simulink model "MAS_180_BO"  (R2018b)
settings: Solver=VariableStepAuto  StartTime=0.0  StopTime=10.0  RelTol=1e-3
values from neighbouring files (symbols this model uses):
  A = sqrt(2/3)*[1 -0.5 -0.5; 0 sqrt(3)/2 -sqrt(3)/2; sqrt(0.5) sqrt(0.5) sqrt(0.5)]    [MAS_EVV_init.m]
  a1 = input('Reponse : ')    [MAS_EVV_init.m]
  Ai = inv(A)    [MAS_EVV_init.m]
  alfa = 3.98e-3    (= 0.00398)    [MAS_EVV_init.m]
  b1 = input('Reponse : ')    [MAS_EVV_init.m]
  Bi = [1/(sigma*Ls) 0 -Msr/(sigma*Ls*Lr) 0; 0 1/(sigma*Ls) 0 -Msr/(sigma*Ls*Lr); -Msr/(sigma*Ls*Lr) 0 1/(sigma*Ls) 0; 0 -Msr/(sigma*Ls*Lr) 0 1/(sigma*Ls) ]    [MAS_EVV_init.m]
  c1 = input('Reponse : ')    [MAS_EVV_init.m]
  d1 = input('Reponse : ')    [MAS_EVV_init.m]
  delta_T = 80    [MAS_EVV_init.m]
  f = (alpha/100)*Pn/(Wn)^2    (= 0.000141076783904)    [MAS_EVV_init.m]    (also in fct_trans.m)
  J = 0.51    [MAS_EVV_init.m]    (also in fct_trans.m)
  Lr = (N2w/2+L1w)/wn    [MAS_EVV_init.m]    (also in fct_trans.m)
  Ls = (N2w/2+L1w)/wn    [MAS_EVV_init.m]    (also in fct_trans.m)
  Msr = L1w/wn    [MAS_EVV_init.m]    (also in fct_trans.m)
  P = 1    [MAS_EVV_init.m]    (also in fct_trans.m)
  R0 = Rr/(1+alfa*delta_T)    [MAS_EVV_init.m]
  Rr = double(R2)    [MAS_EVV_init.m]    (also in fct_trans.m)
  Rs = 0.9*Rr    [MAS_EVV_init.m]    (also in fct_trans.m)
  sigma = 1-(Msr^2)/(Ls*Lr)    [MAS_EVV_init.m]    (also in fct_trans.m)
  to = 1    [MAS_EVV_init.m]
  variable = 1    [MAS_EVV_init.m]
  Vn = Un/sqrt(3)    [MAS_EVV_init.m]    (also in fct_trans.m)
  Wn = 2*pi*Nn/60    (= 309.342156623)    [MAS_EVV_init.m]    (also in fct_trans.m)
  wn = 2*pi*fn    (= 314.159265359)    [MAS_EVV_init.m]    (also in fct_trans.m)
settings Model: Creator=cindyiskandar  LastModifiedBy=cindyiskandar

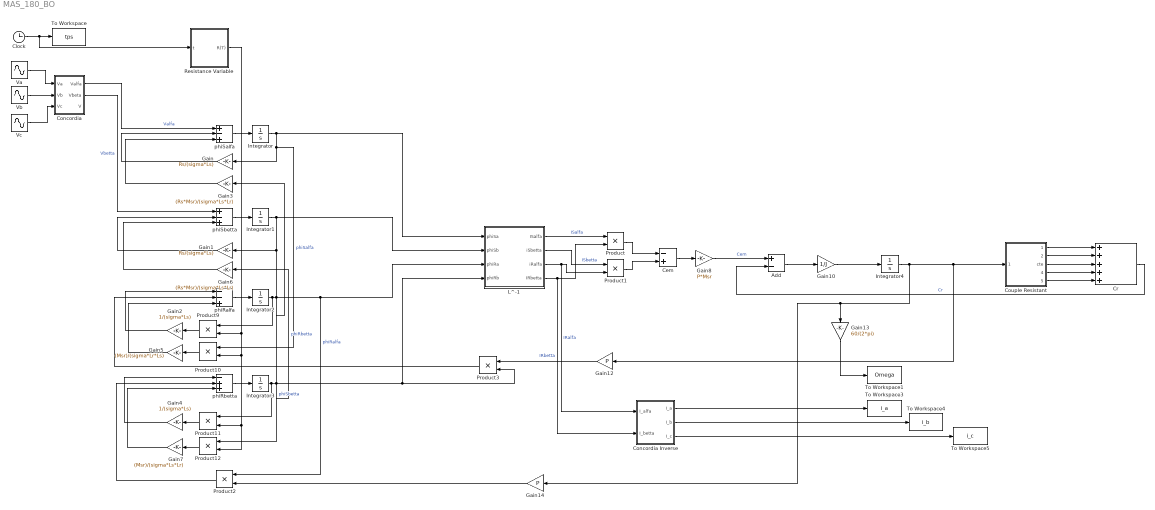
== system MAS_180_BO ==
  Add : Sum  Inputs=+-
  Cem : Sum  Inputs=-+
  Clock : Clock
  "Concordia " : Subsystem
  Concordia Inverse : Subsystem
  Couple Resistant : Subsystem
  "Cr " : Sum  Inputs=+++++
  Gain : Gain  Gain=Rs/(sigma*Ls)
  Gain1 : Gain  Gain=Rs/(sigma*Ls)
  Gain10 : Gain  Gain=1/J
  Gain12 : Gain  Gain=P
  Gain13 : Gain  Gain=60/(2*pi)
  Gain14 : Gain  Gain=P
  Gain2 : Gain  Gain=1/(sigma*Ls)
  Gain3 : Gain  Gain=(Rs*Msr)/(sigma*Ls*Lr)
  Gain4 : Gain  Gain=1/(sigma*Ls)
  Gain5 : Gain  Gain=(Msr)/(sigma*Lr*Ls)
  Gain6 : Gain  Gain=(Rs*Msr)/(sigma*Ls*Lr)
  Gain7 : Gain  Gain=(Msr)/(sigma*Ls*Lr)
  Gain8 : Gain  Gain=P*Msr
  Integrator{,1..4} (5 alike) : Integrator
  "L^-1 " : Subsystem
  Product{,1..3,9..12} (8 alike) : Product
  Resistance Variable : Subsystem
  To Workspace : ToWorkspace  VariableName=tps  SampleTime=-1
      settings: Save2DSignal=2-D array (concatenate along first dimension)
  To Workspace1 : ToWorkspace  VariableName=Omega  SampleTime=-1
      settings: Save2DSignal=2-D array (concatenate along first dimension)
  To Workspace3 : ToWorkspace  VariableName=i_a  SampleTime=-1
      settings: Save2DSignal=2-D array (concatenate along first dimension)
  To Workspace4 : ToWorkspace  VariableName=i_b  SampleTime=-1
      settings: Save2DSignal=2-D array (concatenate along first dimension)
  To Workspace5 : ToWorkspace  VariableName=i_c  SampleTime=-1
      settings: Save2DSignal=2-D array (concatenate along first dimension)
  Va : Sin  Amplitude=Vn*sqrt(2)  Frequency=wn  SampleTime=0
  Vb : Sin  Amplitude=Vn*sqrt(2)  Frequency=wn  Phase=4*pi/3  SampleTime=0
  Vc : Sin  Amplitude=Vn*sqrt(2)  Frequency=wn  Phase=2*pi/3  SampleTime=0
  phiRalfa : Sum  Inputs=--+
  phiRbetta : Sum  Inputs=-++
  phiSalfa : Sum  Inputs=+-+
  phiSbetta : Sum  Inputs=+-+
  wires:
  Product10/1 -> Gain5/1
  Gain13/1 -> To Workspace1/1
  Va/1 -> "Concordia "/1("Va ")
  Cem/1 -> Gain8/1
  Integrator/1 -> Product10/1, Gain/1, "L^-1 "/1(phiSa)  "phiSalfa"
  Gain7/1 -> phiRbetta/3
  Product1/1 -> Cem/2
  phiRalfa/1 -> Integrator2/1
  phiSalfa/1 -> Integrator/1
  Gain10/1 -> Integrator4/1
  Integrator3/1 -> Product11/1, Gain6/1, "L^-1 "/4(phiRb), Product3/2  "phiRbetta"
  Product11/1 -> Gain4/1
  phiSbetta/1 -> Integrator1/1
  Product9/1 -> Gain2/1
  Couple Resistant/3(cte) -> "Cr "/3
  phiRbetta/1 -> Integrator3/1
  Integrator1/1 -> Product12/1, Gain1/1, "L^-1 "/2(phiSb)  "phiSbetta"
  Gain5/1 -> phiRalfa/3
  Gain8/1 -> Add/1  "Cem"
  Integrator4/1 -> Gain14/1, Gain13/1, Gain12/1, Couple Resistant/1(Vitesse)
  Gain4/1 -> phiRbetta/1
  "Concordia "/2("Vbeta ") -> phiSbetta/1  "Vbetta"
  Product12/1 -> Gain7/1
  "Concordia "/1(Valfa) -> phiSalfa/1  "Valfa"
  "L^-1 "/4(IRbetta) -> Concordia Inverse/2(I_betta), Product/2  "IRbetta"
  Gain/1 -> phiSalfa/2
  Gain3/1 -> phiSalfa/3
  Couple Resistant/5(friction) -> "Cr "/5
  Gain1/1 -> phiSbetta/2
  Product3/1 -> phiRalfa/2
  "Cr "/1 -> Add/2  "Cr"
  "L^-1 "/1(ISalfa) -> Product/1  "ISalfa"
  "L^-1 "/3(iRalfa) -> Concordia Inverse/1(I_alfa), Product1/2  "IRalfa"
  Gain2/1 -> phiRalfa/1
  Couple Resistant/4(1/vitesse) -> "Cr "/4
  Integrator2/1 -> Product9/1, Product2/1, "L^-1 "/3(phiRa), Gain3/1  "phiRalfa"
  Product/1 -> Cem/1
  "L^-1 "/2(iSbetta) -> Product1/1  "ISbetta"
  Add/1 -> Gain10/1
  Gain12/1 -> Product3/1
  Concordia Inverse/3(I_c) -> To Workspace5/1
  Couple Resistant/1(vitesse^2) -> "Cr "/1
  Concordia Inverse/1(I_a) -> To Workspace3/1
  Product2/1 -> phiRbetta/2
  Couple Resistant/2(vitesse) -> "Cr "/2
  Concordia Inverse/2(I_b) -> To Workspace4/1
  Gain14/1 -> Product2/2
  Gain6/1 -> phiSbetta/3
  Vb/1 -> "Concordia "/2("Vb ")
  Vc/1 -> "Concordia "/3(Vc)
  Resistance Variable/1(R(T)) -> Product12/2, Product11/2, Product10/2, Product9/2
  Clock/1 -> Resistance Variable/1("t "), To Workspace/1

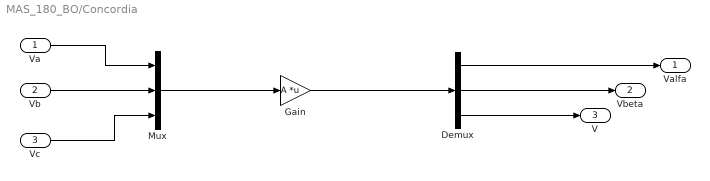
== system MAS_180_BO/Concordia  ==
  "Va " : Inport
  "Vb " : Inport  Port=2
  Vc : Inport  Port=3
  Demux : Demux  Outputs=3
  Gain : Gain  Gain=A  Multiplication=Matrix(K*u) (u vector)
  Mux : Mux  Inputs=3
  Valfa : Outport
  "Vbeta " : Outport  Port=2
  V : Outport  Port=3
  wires:
  Demux/1 -> Valfa/1
  "Va "/1 -> Mux/1
  Mux/1 -> Gain/1
  Gain/1 -> Demux/1
  "Vb "/1 -> Mux/2
  Vc/1 -> Mux/3
  Demux/2 -> "Vbeta "/1
  Demux/3 -> V/1

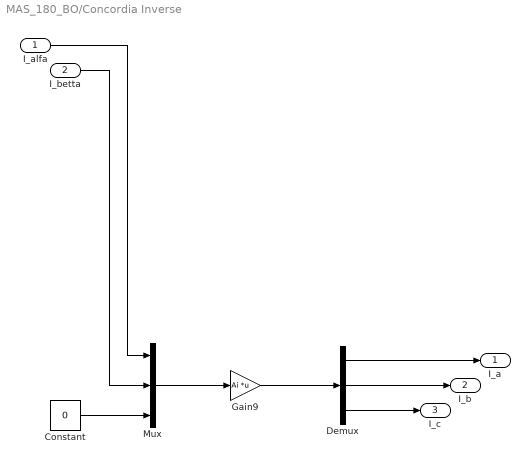
== system MAS_180_BO/Concordia Inverse ==
  I_alfa : Inport
  I_betta : Inport  Port=2
  Constant : Constant  Value=0
  Demux : Demux  Outputs=3
  Gain9 : Gain  Gain=Ai  Multiplication=Matrix(K*u) (u vector)
  Mux : Mux  Inputs=3
  I_a : Outport
  I_b : Outport  Port=2
  I_c : Outport  Port=3
  wires:
  Demux/3 -> I_c/1
  Gain9/1 -> Demux/1
  Demux/1 -> I_a/1
  Demux/2 -> I_b/1
  I_betta/1 -> Mux/2
  I_alfa/1 -> Mux/1
  Mux/1 -> Gain9/1
  Constant/1 -> Mux/3

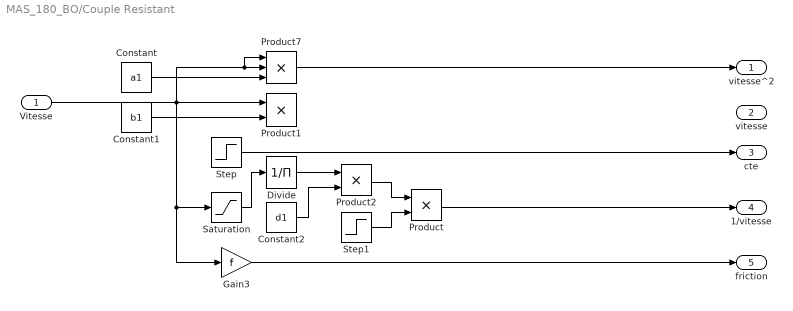
== system MAS_180_BO/Couple Resistant ==
  Vitesse : Inport
  Constant : Constant  Value=a1
  Constant1 : Constant  Value=b1
  Constant2 : Constant  Value=d1
  Divide : Product  Inputs=/
  Gain3 : Gain  Gain=f
  Product : Product
  Product1 : Product
  Product2 : Product
  Product7 : Product  Inputs=3
  Saturation : Saturate  UpperLimit=Wn  LowerLimit=0.01  OutMin=[0.01]  OutMax=[Wn]
  Step : Step  Time=2  After=c1  SampleTime=0
  Step1 : Step  Time=2  SampleTime=0
  vitesse^2 : Outport
  vitesse : Outport  Port=2
  cte : Outport  Port=3
  1/vitesse : Outport  Port=4
  friction : Outport  Port=5
  wires:
  Vitesse/1 -> Product1/1, Product7/2, Product7/1, Gain3/1, Saturation/1
  Step/1 -> cte/1
  Product7/1 -> vitesse^2/1
  Gain3/1 -> friction/1
  Saturation/1 -> Divide/1
  Product/1 -> 1/vitesse/1
  Step1/1 -> Product/2
  Constant/1 -> Product7/3
  Constant1/1 -> Product1/2
  Product2/1 -> Product/1
  Divide/1 -> Product2/1
  Constant2/1 -> Product2/2

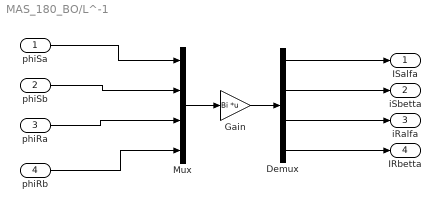
== system MAS_180_BO/L^-1  ==
  phiSa : Inport
  phiSb : Inport  Port=2
  phiRa : Inport  Port=3
  phiRb : Inport  Port=4
  Demux : Demux
  Gain : Gain  Gain=Bi  Multiplication=Matrix(K*u) (u vector)
  Mux : Mux
  ISalfa : Outport
  iSbetta : Outport  Port=2
  iRalfa : Outport  Port=3
  IRbetta : Outport  Port=4
  wires:
  phiRb/1 -> Mux/4
  Demux/4 -> IRbetta/1
  Mux/1 -> Gain/1
  Gain/1 -> Demux/1
  Demux/1 -> ISalfa/1
  phiSa/1 -> Mux/1
  phiRa/1 -> Mux/3
  Demux/3 -> iRalfa/1
  phiSb/1 -> Mux/2
  Demux/2 -> iSbetta/1

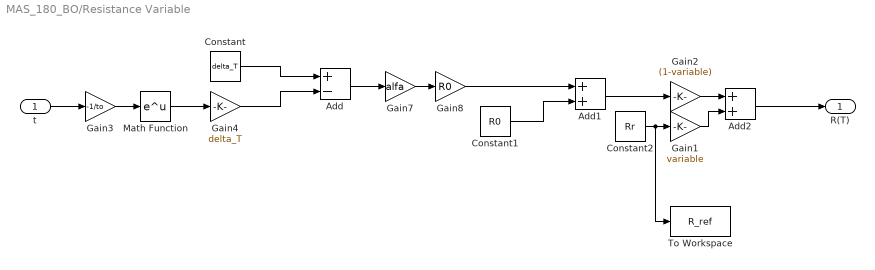
== system MAS_180_BO/Resistance Variable ==
  "t " : Inport
  Add : Sum  Inputs=+-
  Add1 : Sum
  Add2 : Sum
  Constant : Constant  Value=delta_T
  Constant1 : Constant  Value=R0
  Constant2 : Constant  Value=Rr
  Gain1 : Gain  Gain=variable
  Gain2 : Gain  Gain=(1-variable)
  Gain3 : Gain  Gain=-1/to
  Gain4 : Gain  Gain=delta_T
  Gain7 : Gain  Gain=alfa
  Gain8 : Gain  Gain=R0
  Math Function : Math  SaturateOnIntegerOverflow=on
  To Workspace : ToWorkspace  VariableName=R_ref  SampleTime=-1
      settings: Save2DSignal=2-D array (concatenate along first dimension)
  R(T) : Outport
  wires:
  "t "/1 -> Gain3/1
  Gain7/1 -> Gain8/1
  Add1/1 -> Gain2/1
  Gain4/1 -> Add/2
  Gain3/1 -> Math Function/1
  Gain8/1 -> Add1/1
  Constant/1 -> Add/1
  Math Function/1 -> Gain4/1
  Constant1/1 -> Add1/2
  Add/1 -> Gain7/1
  Constant2/1 -> To Workspace/1, Gain1/1
  Gain1/1 -> Add2/2
  Gain2/1 -> Add2/1
  Add2/1 -> R(T)/1
